simulink model "Car_suspension_system"  (R2021a)
settings: Solver=ode45  StartTime=0.0  StopTime=15  RelTol=1e-3
values from neighbouring files (symbols this model uses):
  b = 5500    [Run_car_suspension_system.m]
  k1 = 7500    [Run_car_suspension_system.m]
  k2 = 170000    [Run_car_suspension_system.m]
  M = 700    [Run_car_suspension_system.m]
settings Model: Creator=cop20skj  LastModifiedBy=cop20skj

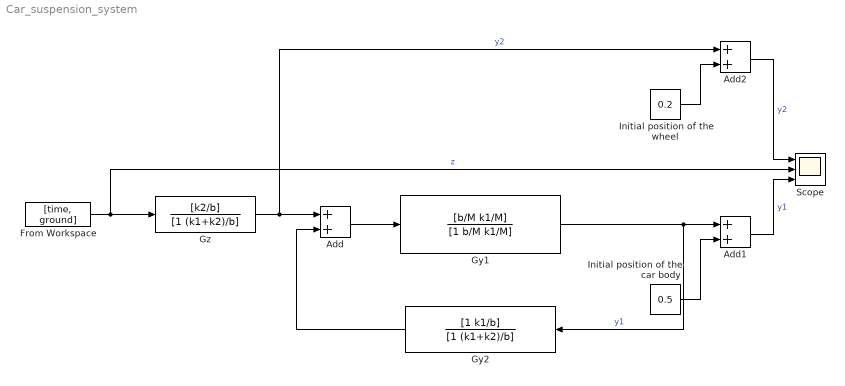
== system Car_suspension_system ==
  Add : Sum
  Add1 : Sum
  Add2 : Sum
  From Workspace : FromWorkspace  VariableName=[time, ground]
  Gy1 : TransferFcn  Numerator=[b/M k1/M]  Denominator=[1 b/M k1/M]
  Gy2 : TransferFcn  Numerator=[1 k1/b]  Denominator=[1 (k1+k2)/b]
  Gz : TransferFcn  Numerator=[k2/b]  Denominator=[1 (k1+k2)/b]
  Initial position of the car body : Constant  Value=0.5
  Initial position of the wheel : Constant  Value=0.2
  Scope : Scope  NumInputPorts=3
  wires:
  From Workspace/1 -> Scope/2, Gz/1  "z"
  Gz/1 -> Add2/1, Add/1  "y2"
  Add/1 -> Gy1/1
  Gy1/1 -> Gy2/1, Add1/1  "y1"
  Gy2/1 -> Add/2
  Initial position of the car body/1 -> Add1/2
  Add1/1 -> Scope/3  "y1"
  Add2/1 -> Scope/1  "y2"
  Initial position of the wheel/1 -> Add2/2
